simulink model "lab1_q11_sim"  (R2025a)
settings: Solver=VariableStepAuto  StartTime=0.0  StopTime=10.0  RelTol=1e-3
values from neighbouring files (symbols this model uses):
  B = 20    [lab1.m]
  J = 1    [lab1.m]
  Ka2 = 19.8    [lab1.m]
  Km = 5    [lab1.m]
  L = 1e-3    (= 0.001)    [lab1.m]
  R = 1    [lab1.m]
settings Model: Creator=alexj  LastModifiedBy=alexj

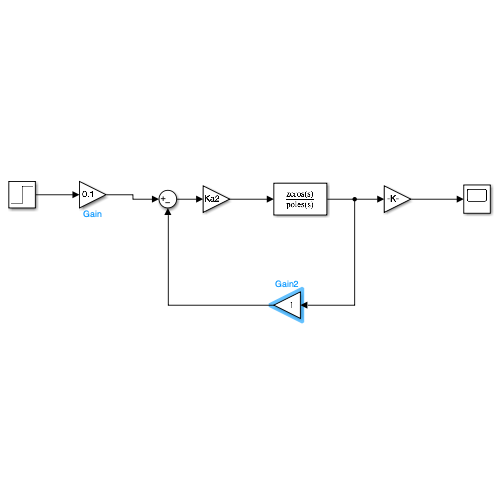
[thumbnail: Simulink's stored preview of the top-level diagram]
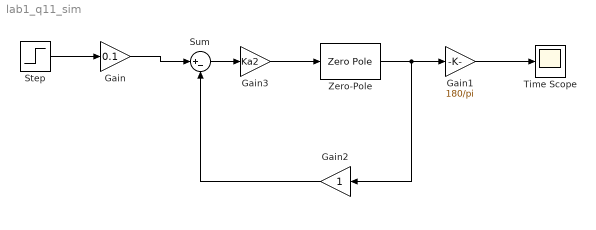
== system lab1_q11_sim ==
  Gain : Gain  Gain=0.1
  Gain1 : Gain  Gain=180/pi
  Gain2 : Gain
  Gain3 : Gain  Gain=Ka2
  Step : Step  SampleTime=0
  Sum : Sum  Inputs=|+-
  Time Scope : Scope
      settings: TimeUnits=Metric (based on Time Span)  YLabel=Amplitude
  Zero-Pole : ZeroPole  Zeros=[]  Poles=[0, -B/J, -R/L]  Gain=Km/(J*L)
  wires:
  Step/1 -> Gain/1
  Gain/1 -> Sum/1
  Zero-Pole/1 -> Gain2/1, Gain1/1
  Gain1/1 -> Time Scope/1
  Gain2/1 -> Sum/2
  Sum/1 -> Gain3/1
  Gain3/1 -> Zero-Pole/1
